simulink model "ResidentialPVArray"  (R2024b)
settings: Solver=FixedStepDiscrete  StartTime=0.0  StopTime=0.8  FixedStep=Ts_Power  RelTol=1e-4
PreLoadFcn:
  | Ts_Power=5e-6;
  | Ts_Control=25e-6;
  | Vf_Diode=0.6;
undefined symbols (not defined in the file or in its folder): DiscIntNeverNeededParam
libraries: spsDiodeLib x7, spsSeriesRLCLoadLib x6, spsPVArrayLib x6, spsVoltageMeasurementLib x5, spsSeriesRLCBranchLib x5, spsCurrentMeasurementLib x4, simulink x4, spsPowerLib x3, spsMeanLib x3, spsStairGeneratorLib x2, spsFirstOrderFilterLib x2, spsPWMGeneratorPulseAveragingLib x2
settings Model: SimulationMode=accelerator  Creator=The MathWorks, Inc.  LastModifiedBy=Jatay
settings SolverCC: AlgebraicLoopSolver=TrustRegion
settings DataIOCC: SaveFormat=StructureWithTime  SaveOutput=off  DSMLogging=off  SaveTime=off  ReturnWorkspaceOutputs=off
settings DebuggingCC: UnconnectedInputMsg=warning  UnconnectedOutputMsg=warning  UnconnectedLineMsg=warning  ArithmeticOperatorsInVariantConditions=warning
settings ModelReferenceCC: EnableRefExpFcnMdlSchedulingChecks=on
settings SFSimCC: CustomCodeUndefinedFunction=UseInterfaceOnly
settings RTWCC: GPUComputeCapability=3.5

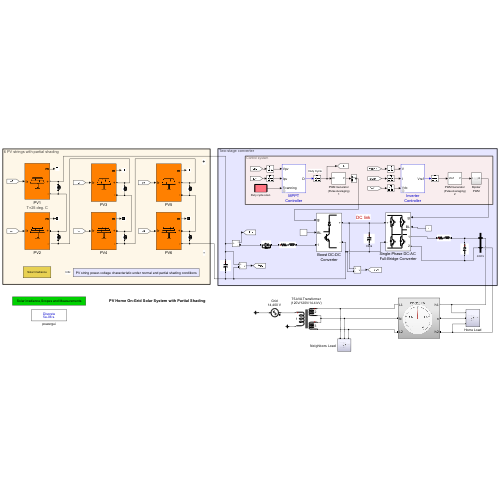
[thumbnail: Simulink's stored preview of the top-level diagram]
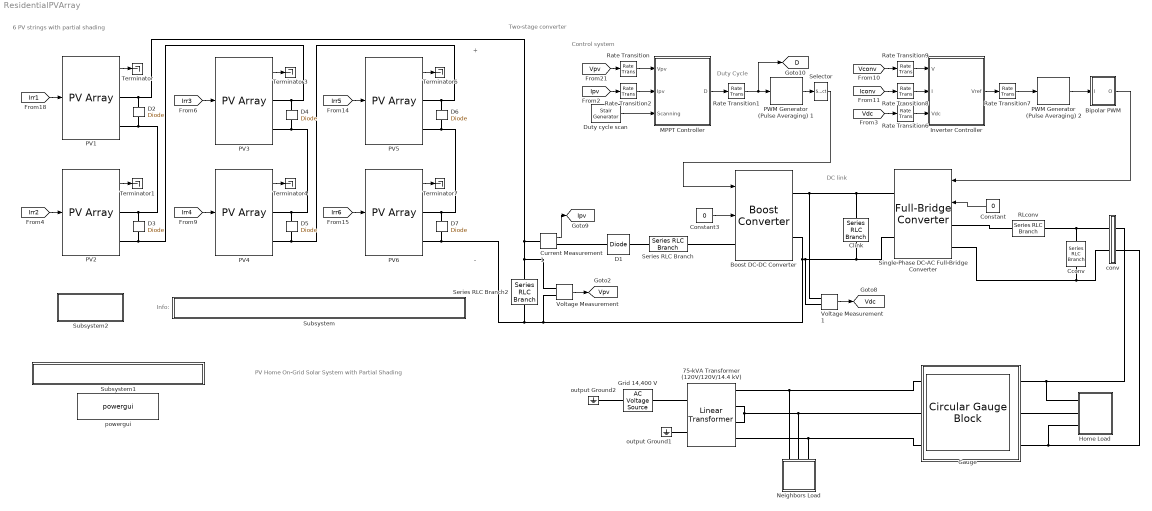
== system ResidentialPVArray ==
  note: Duty Cycle
  note: DC link
  note: Info:
  note: Control system
  note: Two-stage converter
  note: PV Home On-Grid Solar System with Partial Shading
  note: +
  note: 6 PV strings with partial shading
  note: -
  " " : Subsystem
  75-kVA Transformer (120V/120V/14.4 kV) : spsLinearTransformerLib/Linear Transformer  UNITS=pu  NominalPower=[75e3,60]  winding1=[14.4e3 0.01,0.03]  winding2=[120,0.02,0]  ThreeWindings=on  winding3=[120,0.02,0]  RmLm=[100,100]  Measurements=None  DataType=off
  Bipolar PWM : Subsystem
  Boost DC-DC Converter : spsBoostConverterLib/Boost Converter  ModelType=Switching function  Ron=1e-3  Rs=1e6  Cs=inf  Vforward=[0,0]  Ron_Diode=1e-3  Rs_Diode=1e6  Cs_Diode=inf  Vf_Diode=0  Rs_CurrentSource=inf  Ron_ACsource=1e-3
  Cconv : spsSeriesRLCBranchLib/Series RLC Branch  LConnTagsString=__new0  RConnTagsString=__new0  BranchType=C  Resistance=2  Inductance=10e-3  SetiL0=off  InitialCurrent=0  Capacitance=4e-6  Setx0=off  InitialVoltage=0  Measurements=None
  Clink : spsSeriesRLCBranchLib/Series RLC Branch  LConnTagsString=__new0  RConnTagsString=__new0  BranchType=C  Resistance=1e-6  Inductance=1e-3  SetiL0=off  InitialCurrent=0  Capacitance=5.0e-3  Setx0=on  InitialVoltage=400  Measurements=None
  Constant : Constant  Value=0
  Constant3 : Constant  Value=0
  Current Measurement1 : spsCurrentMeasurementLib/Current Measurement  PhasorSimulation=off  OutputType=Complex  PSBequivalent=0
  D{1..7} (7 alike) : spsDiodeLib/Diode  Ron=1e-3  Lon=0  Vf=Vf_Diode  IC=0  UseSnubber=0  Rs=1e6  Cs=inf  Measurements=off
  Duty cycle scan : spsStairGeneratorLib/Stair Generator  t=[0,0.40, 0.41]  e=[0, 1, 0]  Ts=Ts_Control
  Gauge : CircularGaugeBlock  ScaleMin=-3  ScaleMax=3  TickInterval=1.5
  Grid 14,400 V : spsACVoltageSourceLib/AC Voltage Source  Description=source block  Amplitude=14400*sqrt(2)  Phase=0  Frequency=60  SampleTime=0  Measurements=None  BusType=swing  Pref=10e3  Qref=0  Qmin=-inf  Qmax=+inf
      settings: AttributesFormatString=\n
  Home Load : Subsystem
  Inverter Controller : Subsystem  mask(Inverter Control){Pnom=2500, Fnom=60, Vnom_ac=240, Vnom_dc=400, Kp_VDCreg=10, Ki_VDCreg=1000, Kp_Ireg=0.3, Ki_Ireg=20, RLff=[ 0.003, 0.3], Ts=Ts_Control}
      mask prompts: Pnom "Power (VA)"; Fnom "Frequency (Hz)"; Vnom_ac "AC voltage (Vrms)"; Vnom_dc "DC voltage (V)"; Kp_VDCreg "Proportional gain"; Ki_VDCreg "Integral gain"; Kp_Ireg "Proportional gain"; Ki_Ireg "Integral gain"; RLff "Feedforward Values [Rff Lff] (pu)"; Ts "Control sample time:"
      mask help: Control system for a 2.5 kW Grid-Connected Inverter
      mask init:
      | Rff=RLff(1);
      | Lff=RLff(2);
      | Limits_Ireg=[1.5, -1.5];
      | Limits_VDCreg=[1.5, -1.5];
      | Limits_Preg=[1.5, -1.5];
      | Limits_Qreg=[1.5, -1.5];
      mask DialogControl Container4 Prompt: Nominal Values:
      mask DialogControl Container8 Prompt: Voltage regulator:
      mask DialogControl Container6 Prompt: Current regulators:
      mask DialogControl Ts1 Prompt: Sample time (s)
  MPPT Controller : Subsystem  mask(MPPT Controller - Perturb and Observe algorithm (PandO)){Dinit=0.39, Dlimits=[0.85, 0.30], deltaD=50e-6, Fc=1000, ScanDuration=0.25, Ts=Ts_Control}
      mask prompts: Dinit "Duty cycle (D) initial value"; Dlimits "D limits [Upper, Lower]"; deltaD "Increment value for PandO algorithm"; Fc "Measurement filter cutoff frequency (Hz)"; ScanDuration "Scanning mode duration (s)"; Ts "Sample time (s)"
      mask init:
      | Dmax=Dlimits(1);
      | Dmin=Dlimits(2);
      | SampleTime=Ts;
      | DeltaD_Scan=(Dmax-Dmin)*Ts/ScanDuration;
  Neighbors Load : Subsystem
  PV1 : spsPVArrayLib/PV Array  Npar=1  Nser=1  PlotType=array @ 25 deg.C & specified irradiances  S_vec=[ 1000 250]  Temp_C_vec="[ 45 25  ]"  ModuleName=User-defined  PlotWhenSelected=off  Pm=400.316  Ncell=72  Voc=49.3  Isc=10.47  Vm=40.6  Im=9.86  beta_Voc_pc=-0.2600  alpha_Isc_pc=0.03  beta_Voc=-0.12818  alpha_Isc=0.003141  IL=10.5166  I0=5.8445e-12  nI=0.94527  Rsh=194.9682  Rs=0.32878  RobustModel=on  RobustCellTemperature=25  BAL=on  Tc=1e-6  Tfilter=5e-5
      settings: AttributesFormatString=T=%<RobustCellTemperature> deg. C
  PV{2..6} (5 alike) : spsPVArrayLib/PV Array  Npar=1  Nser=1  PlotType=array @ 1000 W/m2 & specified temperatures  S_vec=[ 1000 250]  Temp_C_vec="[ 45 25  ]"  ModuleName=User-defined  PlotWhenSelected=off  Pm=400.316  Ncell=72  Voc=49.3  Isc=10.47  Vm=40.6  Im=9.86  beta_Voc_pc=-0.2600  alpha_Isc_pc=0.03  beta_Voc=-0.12818  alpha_Isc=0.003141  IL=10.5166  I0=5.8445e-12  nI=0.94527  Rsh=194.9682  Rs=0.32878  RobustModel=on  RobustCellTemperature=25  BAL=on  Tc=1e-6  Tfilter=5e-5
  PWM Generator (Pulse Averaging) 1 : spsPWMGeneratorPulseAveragingLib/PWM Generator (Pulse Averaging)  GeneratorType=Two-quadrant  Fc=20e3  InitialPhase=90  Ts=Ts_Power
  PWM Generator (Pulse Averaging) 2 : spsPWMGeneratorPulseAveragingLib/PWM Generator (Pulse Averaging)  GeneratorType=Full-bridge, single phase  Fc=20e3  InitialPhase=90  Ts=Ts_Power
  RLconv : spsSeriesRLCBranchLib/Series RLC Branch  LConnTagsString=__new0  RConnTagsString=__new0  BranchType=RL  Resistance=75e-3  Inductance=20e-3  SetiL0=off  InitialCurrent=0  Capacitance=1e-6  Setx0=off  InitialVoltage=0  Measurements=None
  Rate Transition{,2,6,8..9} (5 alike) : RateTransition  OutPortSampleTime=Ts_Control
  Rate Transition1 : RateTransition  OutPortSampleTime=Ts_Power
  Rate Transition7 : RateTransition  OutPortSampleTime=Ts_Power
  Selector : Selector  InputPortWidth=2  IndexOptions=Index vector (dialog)  Indices=1  OutputSizes=1
  Series RLC Branch : spsSeriesRLCBranchLib/Series RLC Branch  LConnTagsString=__new0  RConnTagsString=__new0  BranchType=RL  Resistance=20e-3  Inductance=20e-3  SetiL0=off  InitialCurrent=0  Capacitance=1e-6  Setx0=off  InitialVoltage=0  Measurements=None
  Series RLC Branch2 : spsSeriesRLCBranchLib/Series RLC Branch  LConnTagsString=__new0  RConnTagsString=__new0  BranchType=C  Resistance=10e-3  Inductance=10e-3  SetiL0=off  InitialCurrent=0  Capacitance=10e-6  Setx0=off  InitialVoltage=0  Measurements=None
  Single-Phase DC-AC Full-Bridge Converter : spsFullBridgeConverterLib/Full-Bridge Converter  ModelType=Switching function  Ron=1e-3  Rs=1e6  Cs=inf  Vforward=[0,0]  Ron_Diode=1e-3  Rs_Diode=1e6  Cs_Diode=inf  Vf_Diode=0  Rs_CurrentSource=inf  Ron_ACsource=1e-3
  Subsystem : Subsystem
      mask Display: disp('PV string power-voltage characteristic under normal and partial shading conditions')
  Subsystem1 : Subsystem
      mask Display: disp('Solar irradiance,Scopes and Measurements')
  Subsystem2 : Subsystem
      mask Display: disp('Solar Irradiance')
  Terminator{,1,3..4,6..7} (6 alike) : Terminator
  Voltage Measurement : spsVoltageMeasurementLib/Voltage Measurement  PhasorSimulation=off  OutputType=Complex  PSBequivalent=0
  Voltage Measurement1 : spsVoltageMeasurementLib/Voltage Measurement  PhasorSimulation=off  OutputType=Complex  PSBequivalent=0
  conv : Subsystem
  output Ground1 : spsGroundLib/Ground  LConnTagsString=a
  output Ground2 : spsGroundLib/Ground  LConnTagsString=a
  powergui : spspowerguiLib/powergui  Priority=2  SimulationMode=Discrete  SampleTime=Ts_Power  frequency=60  Iterations=50  frequencyindice=0  Pbase=100e6  ErrMax=1e-4  UnitsV=kV  UnitsW=MW  buscounter=0  FunctionMessages=off  echomessages=off  EnableUseOfTLC=off  CurrentSourceSwitches=off  DisableSnubberDevices=off  DisableRonSwitches=off  DisableVfSwitches=off  DisplayEquations=off  AutomaticDiscreteSolvers=off  SolverType=Tustin/Backward Euler (TBE)  Interpol=off  ExternalGateDelay=off  methode=off  Ts=0  x0status=blocks  SPID=off  SwTol=0  HookPort=off  NonlinearTolerance=1e-4  nMaxIteration=100  ContinueOnMaxIteration=on  RestoreLinks=warning  ResistiveCurrentMeasurement=off  Frange=[0:2:500]  Ylog=off  Xlog=off  ShowGrid=off  save=off  variable=ZData  structure=Scope_VIgrid  ZoomFFT=off  StartTime=0.27  cycles=1  DisplayStyle=1  fundamental=60  FreqAxis=off  MaxFrequency=25000  frequencyindicesteady=1  RmsSteady=1  display=off
  tag scope: D=global, Ipv=global, Vdc=global, Vpv=global
  wires:
  [Irr1] -> PV1/1
  MPPT Controller/1(D) -> Rate Transition1/1
  PV1/1 -> Terminator/1
  [Irr2] -> PV2/1
  PV2/1 -> Terminator1/1
  [Irr3] -> PV3/1
  PV3/1 -> Terminator3/1
  PV4/1 -> Terminator4/1
  [Irr4] -> PV4/1
  PV6/1 -> Terminator7/1
  PV5/1 -> Terminator6/1
  [Irr6] -> PV6/1
  [Irr5] -> PV5/1
  Voltage Measurement/1 -> [Vpv]
  Constant3/1 -> Boost DC-DC Converter/2
  Duty cycle scan/1 -> MPPT Controller/3(Scanning)
  [Ipv] -> Rate Transition2/1
  [Vpv] -> Rate Transition/1
  Rate Transition/1 -> MPPT Controller/1(Vpv)
  Rate Transition2/1 -> MPPT Controller/2(Ipv)
  [Vconv] -> Rate Transition9/1
  [Vdc] -> Rate Transition6/1
  [Iconv] -> Rate Transition8/1
  Rate Transition6/1 -> Inverter Controller/3(Vdc)
  Rate Transition8/1 -> Inverter Controller/2(I)
  Rate Transition9/1 -> Inverter Controller/1(V)
  Voltage Measurement1/1 -> [Vdc]
  Constant/1 -> Single-Phase DC-AC Full-Bridge Converter/2
  Current Measurement1/1 -> [Ipv]
  Rate Transition7/1 -> PWM Generator (Pulse Averaging) 2/1
  Inverter Controller/1(Vref) -> Rate Transition7/1
  Rate Transition1/1 -> PWM Generator (Pulse Averaging) 1/1, [D]
  Selector/1 -> Boost DC-DC Converter/1
  PWM Generator (Pulse Averaging) 1/1 -> Selector/1
  PWM Generator (Pulse Averaging) 2/1 -> Bipolar PWM/1(I)
  Bipolar PWM/1(O) -> Single-Phase DC-AC Full-Bridge Converter/1
  connections:
  PV5/RConn1 -- D5/LConn1 -- PV4/RConn2 -- D6/RConn1
  D2/LConn1 -- D3/RConn1 -- PV2/RConn1 -- PV1/RConn2
  D4/RConn1 -- D3/LConn1 -- PV2/RConn2 -- PV3/RConn1
  D4/LConn1 -- D5/RConn1 -- PV4/RConn1 -- PV3/RConn2
  D6/LConn1 -- D7/RConn1 -- PV6/RConn1 -- PV5/RConn2
  D1/RConn1 -- Series RLC Branch/LConn1
  Series RLC Branch/RConn1 -- Boost DC-DC Converter/LConn1
  D7/LConn1 -- PV6/RConn2 -- Series RLC Branch2/RConn1 -- Voltage Measurement/LConn2 -- Clink/RConn1 -- Single-Phase DC-AC Full-Bridge Converter/RConn2 -- Voltage Measurement1/LConn2 -- Boost DC-DC Converter/RConn2
  Clink/LConn1 -- Single-Phase DC-AC Full-Bridge Converter/RConn1 -- Voltage Measurement1/LConn1 -- Boost DC-DC Converter/RConn1
  Current Measurement1/RConn1 -- D1/LConn1
  75-kVA Transformer (120V/120V/14.4 kV)/RConn2 -- " "/RConn2 -- Neighbors Load/LConn2 -- 75-kVA Transformer (120V/120V/14.4 kV)/RConn3
  output Ground2/LConn1 -- Grid 14,400 V/LConn1
  Single-Phase DC-AC Full-Bridge Converter/LConn1 -- RLconv/LConn1
  Grid 14,400 V/RConn1 -- 75-kVA Transformer (120V/120V/14.4 kV)/LConn1
  Single-Phase DC-AC Full-Bridge Converter/LConn2 -- Cconv/RConn1 -- conv/LConn2
  RLconv/RConn1 -- Cconv/LConn1 -- conv/LConn1
  Voltage Measurement/LConn1 -- D2/RConn1 -- PV1/RConn1 -- Current Measurement1/LConn1 -- Series RLC Branch2/LConn1
  " "/RConn1 -- Neighbors Load/LConn1 -- 75-kVA Transformer (120V/120V/14.4 kV)/RConn1
  Home Load/LConn1 -- conv/RConn1 -- " "/LConn1
  conv/RConn2 -- Home Load/LConn3 -- " "/LConn3
  " "/RConn3 -- Neighbors Load/LConn3 -- 75-kVA Transformer (120V/120V/14.4 kV)/RConn4
  Home Load/LConn2 -- " "/LConn2
  output Ground1/LConn1 -- 75-kVA Transformer (120V/120V/14.4 kV)/LConn2

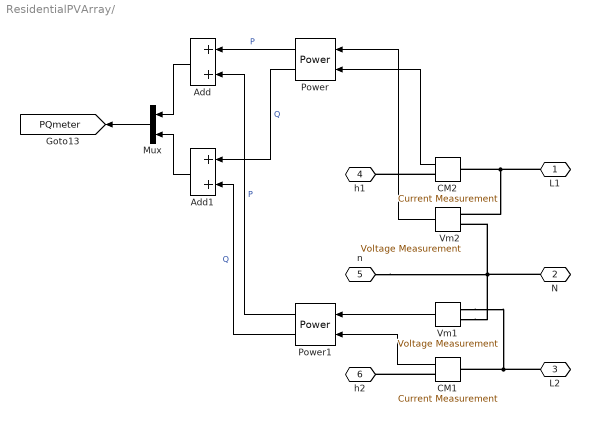
== system ResidentialPVArray/  ==
  Add : Sum
  Add1 : Sum
  CM1 : spsCurrentMeasurementLib/Current Measurement  PhasorSimulation=off  OutputType=Complex  PSBequivalent=0
  CM2 : spsCurrentMeasurementLib/Current Measurement  PhasorSimulation=off  OutputType=Complex  PSBequivalent=0
  Mux : Mux  Inputs=2
  Power : spsPowerLib/Power  Freq=60  Vinit=[120*sqrt(2), 0]*0  Iinit=[10*sqrt(2), 10]*0  Ts=Ts_Power
  Power1 : spsPowerLib/Power  Freq=60  Vinit=[120*sqrt(2), 0]*0  Iinit=[10*sqrt(2), 10]*0  Ts=Ts_Power
  Vm1 : spsVoltageMeasurementLib/Voltage Measurement  PhasorSimulation=off  OutputType=Complex  PSBequivalent=0
  Vm2 : spsVoltageMeasurementLib/Voltage Measurement  PhasorSimulation=off  OutputType=Complex  PSBequivalent=0
  L1 : PMIOPort  Side=Right
  N : PMIOPort  Port=2  Side=Right
  L2 : PMIOPort  Port=3  Side=Right
  h1 : PMIOPort  Port=4  Side=Left
  n : PMIOPort  Port=5  Side=Left
  h2 : PMIOPort  Port=6  Side=Left
  tag scope: PQmeter=global
  wires:
  Vm2/1 -> Power/1
  CM2/1 -> Power/2
  Vm1/1 -> Power1/1
  CM1/1 -> Power1/2
  Power/1 -> Add/1  "P"
  Power1/1 -> Add/2  "P"
  Add/1 -> Mux/1
  Power/2 -> Add1/1  "Q"
  Power1/2 -> Add1/2  "Q"
  Add1/1 -> Mux/2
  Mux/1 -> [PQmeter]
  connections:
  Vm1/LConn2 -- N/RConn1 -- n/RConn1 -- Vm2/LConn2
  Vm2/LConn1 -- L1/RConn1 -- CM2/LConn1
  CM2/RConn1 -- h1/RConn1
  L2/RConn1 -- Vm1/LConn1 -- CM1/LConn1
  CM1/RConn1 -- h2/RConn1

== system ResidentialPVArray/Bipolar PWM ==
  I : Inport
  Demux : Demux
  Mux : Mux
  Terminator : Terminator
  Terminator1 : Terminator
  O : Outport  VectorParamsAs1DForOutWhenUnconnected=off
  wires:
  Demux/4 -> Terminator1/1
  Demux/3 -> Terminator/1
  Demux/2 -> Mux/2, Mux/3
  Demux/1 -> Mux/1, Mux/4
  I/1 -> Demux/1
  Mux/1 -> O/1

== system ResidentialPVArray/Home Load ==
  HomeLoad 120V_1 : spsSeriesRLCLoadLib/Series RLC Load  LConnTagsString=a  RConnTagsString=__new0  NominalVoltage=120  NominalFrequency=60  ActivePower=600  InductivePower=0  CapacitivePower=0  Setx0=off  InitialVoltage=0  SetiL0=off  InitialCurrent=0  Measurements=None  LoadType=constant Z
  HomeLoad 120V_2 : spsSeriesRLCLoadLib/Series RLC Load  LConnTagsString=a  RConnTagsString=__new0  NominalVoltage=120  NominalFrequency=60  ActivePower=400  InductivePower=0  CapacitivePower=0  Setx0=off  InitialVoltage=0  SetiL0=off  InitialCurrent=0  Measurements=None  LoadType=constant Z
  HomeLoad 240V : spsSeriesRLCLoadLib/Series RLC Load  LConnTagsString=a  RConnTagsString=__new0  NominalVoltage=240  NominalFrequency=60  ActivePower=1.5e3  InductivePower=250  CapacitivePower=0  Setx0=off  InitialVoltage=0  SetiL0=off  InitialCurrent=0  Measurements=None  LoadType=constant Z
  R : PMIOPort  Side=Left
  W : PMIOPort  Port=2  Side=Left
  B : PMIOPort  Port=3  Side=Left
  connections:
  HomeLoad 120V_1/RConn1 -- R/RConn1 -- HomeLoad 240V/RConn1
  HomeLoad 120V_2/RConn1 -- W/RConn1 -- HomeLoad 120V_1/LConn1
  HomeLoad 120V_2/LConn1 -- B/RConn1 -- HomeLoad 240V/LConn1

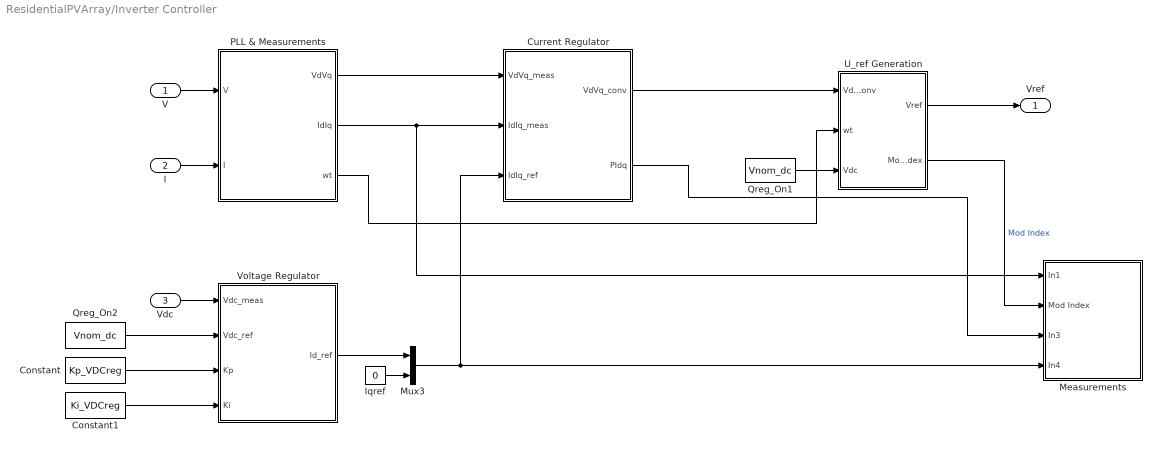
== system ResidentialPVArray/Inverter Controller ==
  V : Inport  PortDimensions=1
  I : Inport  Port=2  PortDimensions=1
  Vdc : Inport  Port=3  PortDimensions=1
  Constant : Constant  Value=Kp_VDCreg  SampleTime=Ts
  Constant1 : Constant  Value=Ki_VDCreg  SampleTime=Ts
  Current Regulator : Subsystem
  Iqref : Constant  Value=0  SampleTime=Ts
  Measurements : Subsystem
  Mux3 : Mux  Inputs=2
  PLL & Measurements : Subsystem
  Qreg_On1 : Constant  Value=Vnom_dc
  Qreg_On2 : Constant  Value=Vnom_dc
  "U_ref Generation " : Subsystem
  Voltage Regulator : Subsystem
  Vref : Outport  VectorParamsAs1DForOutWhenUnconnected=off
  wires:
  Constant/1 -> Voltage Regulator/3(Kp)
  Mux3/1 -> Current Regulator/3(IdIq_ref), Measurements/4(In4)
  V/1 -> PLL & Measurements/1(V)
  Qreg_On2/1 -> Voltage Regulator/2(Vdc_ref)
  PLL & Measurements/2(IdIq) -> Measurements/1(In1), Current Regulator/2(IdIq_meas)
  Voltage Regulator/1(Id_ref) -> Mux3/1
  Constant1/1 -> Voltage Regulator/4(Ki)
  Iqref/1 -> Mux3/2
  I/1 -> PLL & Measurements/2(I)
  Vdc/1 -> Voltage Regulator/1(Vdc_meas)
  PLL & Measurements/1(VdVq) -> Current Regulator/1(VdVq_meas)
  "U_ref Generation "/1(Vref) -> Vref/1
  PLL & Measurements/3(wt) -> "U_ref Generation "/2(wt)
  Qreg_On1/1 -> "U_ref Generation "/3(Vdc)
  Current Regulator/1(VdVq_conv) -> "U_ref Generation "/1(VdVq_conv)
  "U_ref Generation "/2(ModIndex) -> Measurements/2(Mod Index)  "Mod Index"
  Current Regulator/2(PIdq) -> Measurements/3(In3)

== system ResidentialPVArray/MPPT Controller ==
  note: D = 1 - Vsrc/Vdc
  Vpv : Inport
  Ipv : Inport  Port=2
  Scanning : Inport  Port=3  PortDimensions=1
  First-Order Filter : spsFirstOrderFilterLib/First-Order Filter  FilterType=Lowpass  Tc=1/Fc  Ts=Ts  Initialize=off  Vac_Init=[0, 0, 60]  Vdc_Init=0  PlotResponse=off  FreqRange="[0,  200,  1]"
  First-Order Filter1 : spsFirstOrderFilterLib/First-Order Filter  FilterType=Lowpass  Tc=1/Fc  Ts=Ts  Initialize=off  Vac_Init=[0, 0, 60]  Vdc_Init=0  PlotResponse=off  FreqRange="[0,  200,  1]"
  MPPT Control : MATLAB Function  TreatAsAtomicUnit=on
  D : Outport  OutDataTypeStr=double  PortDimensions=1  VectorParamsAs1DForOutWhenUnconnected=off
  wires:
  First-Order Filter1/1 -> MPPT Control/2(I)
  First-Order Filter/1 -> MPPT Control/1(V)
  Ipv/1 -> First-Order Filter1/1
  Vpv/1 -> First-Order Filter/1
  MPPT Control/1(D) -> D/1
  Scanning/1 -> MPPT Control/3(Scan_On)

== system ResidentialPVArray/Neighbors Load ==
  Load 120V_1 : spsSeriesRLCLoadLib/Series RLC Load  LConnTagsString=a  RConnTagsString=__new0  NominalVoltage=120  NominalFrequency=60  ActivePower=7e3  InductivePower=0  CapacitivePower=0  Setx0=off  InitialVoltage=0  SetiL0=off  InitialCurrent=0  Measurements=None  LoadType=constant Z
  Load 120V_2 : spsSeriesRLCLoadLib/Series RLC Load  LConnTagsString=a  RConnTagsString=__new0  NominalVoltage=120  NominalFrequency=60  ActivePower=4e3  InductivePower=0  CapacitivePower=0  Setx0=off  InitialVoltage=0  SetiL0=off  InitialCurrent=0  Measurements=None  LoadType=constant Z
  Load 240V : spsSeriesRLCLoadLib/Series RLC Load  LConnTagsString=a  RConnTagsString=__new0  NominalVoltage=240  NominalFrequency=60  ActivePower=15e3  InductivePower=2000  CapacitivePower=0  Setx0=off  InitialVoltage=0  SetiL0=off  InitialCurrent=0  Measurements=None  LoadType=constant Z
  R : PMIOPort  Side=Left
  W : PMIOPort  Port=2  Side=Left
  B : PMIOPort  Port=3  Side=Left
  connections:
  B/RConn1 -- Load 120V_2/LConn1 -- Load 240V/LConn1
  W/RConn1 -- Load 120V_2/RConn1 -- Load 120V_1/LConn1
  R/RConn1 -- Load 120V_1/RConn1 -- Load 240V/RConn1

== system ResidentialPVArray/Subsystem ==
  note: 6 * LG Electronics Inc. LG400N2W-A5

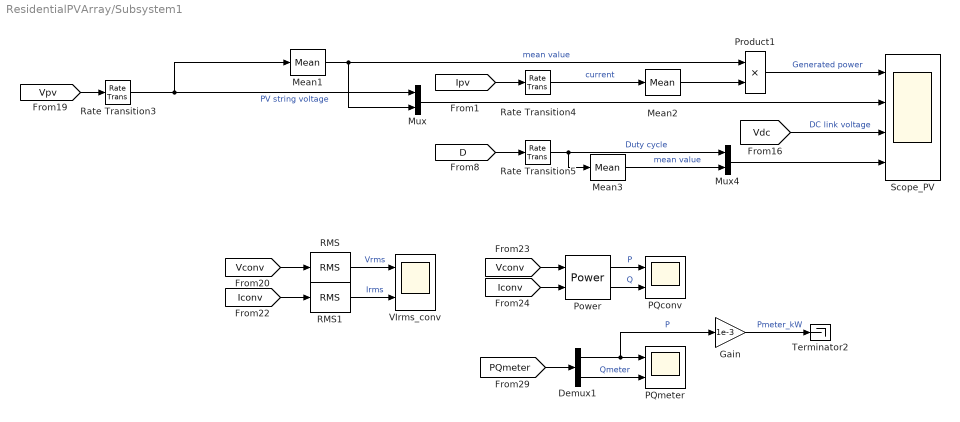
== system ResidentialPVArray/Subsystem1 ==
  Demux1 : Demux  Outputs=2
  Gain : Gain  Gain=1e-3
  Mean1 : spsMeanLib/Mean  Freq=60  Vinit=250  Ts=Ts_Control
  Mean2 : spsMeanLib/Mean  Freq=60  Vinit=10  Ts=Ts_Control
  Mean3 : spsMeanLib/Mean  Freq=60  Vinit=0.4  Ts=Ts_Control
  Mux : Mux  Inputs=2
  Mux4 : Mux  Inputs=2
  PQconv : Scope  NumInputPorts=2
  PQmeter : Scope  NumInputPorts=2
  Power : spsPowerLib/Power  Freq=60  Vinit=[240*sqrt(2), 0]  Iinit=[10*sqrt(2), 10]  Ts=Ts_Power
  Product1 : Product
  RMS : spsRMSLib/RMS  TrueRMS=on  Freq=60  RMSInit=240  Ts=Ts_Power
  RMS1 : spsRMSLib/RMS  TrueRMS=on  Freq=60  RMSInit=10  Ts=Ts_Power
  Rate Transition3 : RateTransition  OutPortSampleTime=Ts_Control
  Rate Transition4 : RateTransition  OutPortSampleTime=Ts_Control
  Rate Transition5 : RateTransition  OutPortSampleTime=Ts_Control
  Scope_PV : Scope  NumInputPorts=4
  Terminator2 : Terminator
  VIrms_conv : Scope  NumInputPorts=2
  wires:
  Gain/1 -> Terminator2/1  "Pmeter_kW"
  [D] -> Rate Transition5/1
  Rate Transition5/1 -> Mean3/1, Mux4/1  "Duty cycle"
  Mean3/1 -> Mux4/2  "mean value"
  Mux4/1 -> Scope_PV/4
  Demux1/2 -> PQmeter/2  "Qmeter"
  [PQmeter] -> Demux1/1
  Demux1/1 -> PQmeter/1, Gain/1  "P"
  [Vconv] -> Power/1
  [Iconv] -> Power/2
  [Iconv] -> RMS1/1
  [Vconv] -> RMS/1
  RMS1/1 -> VIrms_conv/2  "Irms"
  Power/2 -> PQconv/2  "Q"
  Power/1 -> PQconv/1  "P"
  RMS/1 -> VIrms_conv/1  "Vrms"
  [Vdc] -> Scope_PV/3  "DC link voltage"
  Product1/1 -> Scope_PV/1  "Generated power"
  Mux/1 -> Scope_PV/2
  Rate Transition4/1 -> Mean2/1  "current"
  Rate Transition3/1 -> Mean1/1, Mux/1  "PV string voltage"
  Mean2/1 -> Product1/2
  Mean1/1 -> Mux/2, Product1/1  "mean value"
  [Ipv] -> Rate Transition4/1
  [Vpv] -> Rate Transition3/1

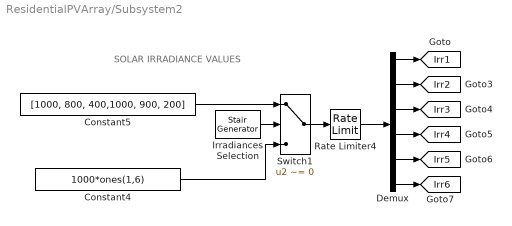
== system ResidentialPVArray/Subsystem2 ==
  note: SOLAR IRRADIANCE VALUES
  Constant4 : Constant  Value=1000*ones(1,6)
  Constant5 : Constant  Value=[1000, 800, 400,1000, 900, 200]
  Demux : Demux  Outputs=6
  Irradiances Selection : spsStairGeneratorLib/Stair Generator  t=[0,0.3, 1.3]  e=[0, 1, 0]  Ts=Ts_Power
  Rate Limiter4 : RateLimiter  RisingSlewLimit=1000*60  FallingSlewLimit=-1000*60  SampleTimeMode=inherited  InitialCondition=1000
  Switch1 : Switch  Criteria=u2 ~= 0  SaturateOnIntegerOverflow=off  InputSameDT=off
  tag scope: Irr1=global, Irr2=global, Irr3=global, Irr4=global, Irr5=global, Irr6=global
  wires:
  Constant5/1 -> Switch1/1
  Demux/5 -> [Irr5]
  Constant4/1 -> Switch1/3
  Irradiances Selection/1 -> Switch1/2
  Rate Limiter4/1 -> Demux/1
  Demux/1 -> [Irr1]
  Switch1/1 -> Rate Limiter4/1
  Demux/3 -> [Irr3]
  Demux/6 -> [Irr6]
  Demux/2 -> [Irr2]
  Demux/4 -> [Irr4]

== system ResidentialPVArray/conv ==
  CM2 : spsCurrentMeasurementLib/Current Measurement  PhasorSimulation=off  OutputType=Complex  PSBequivalent=0
  Vm2 : spsVoltageMeasurementLib/Voltage Measurement  PhasorSimulation=off  OutputType=Complex  PSBequivalent=0
  A : PMIOPort  Side=Left
  B : PMIOPort  Port=2  Side=Left
  a : PMIOPort  Port=3  Side=Right
  b : PMIOPort  Port=4  Side=Right
  tag scope: Iconv=global, Vconv=global
  wires:
  CM2/1 -> [Iconv]
  Vm2/1 -> [Vconv]
  connections:
  CM2/RConn1 -- a/RConn1
  CM2/LConn1 -- A/RConn1 -- Vm2/LConn1
  B/RConn1 -- b/RConn1 -- Vm2/LConn2

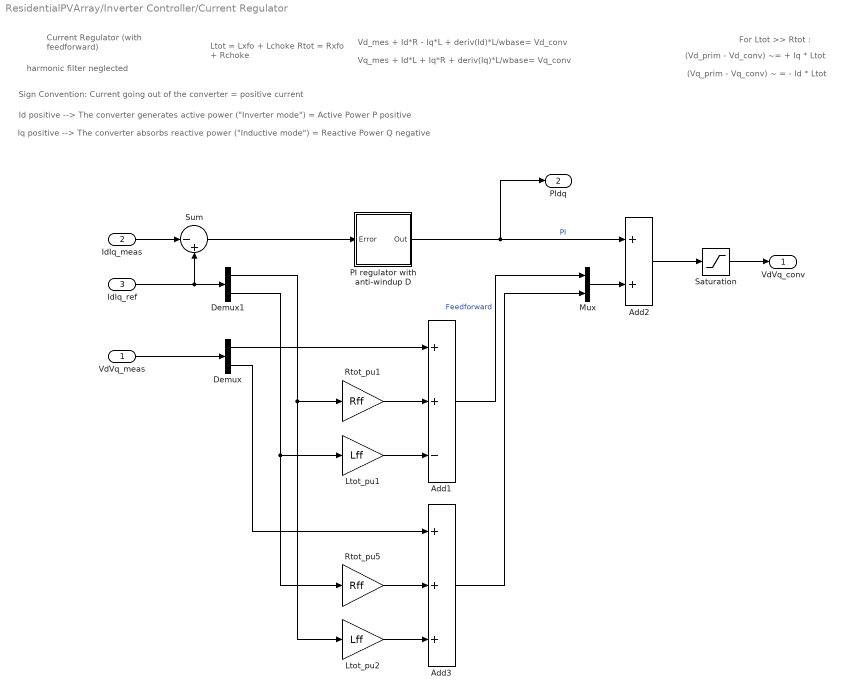
== system ResidentialPVArray/Inverter Controller/Current Regulator ==
  note: harmonic filter neglected
  note: Vd_mes + Id*R - Iq*L + deriv(Id)*L/wbase= Vd_conv
  note: Vq_mes + Id*L + Iq*R + deriv(Iq)*L/wbase= Vq_conv
  note: Current Regulator
      | (with feedforward)
  note: Sign Convention: Current going out of the converter = positive current
  note: Iq positive --> The converter absorbs reactive power ("Inductive mode") = Reactive Power Q negative
  note: Id positive --> The converter generates active power ("Inverter mode") = Active Power P positive
  note: Ltot = Lxfo + Lchoke
      | Rtot = Rxfo + Rchoke
  note: (Vd_prim - Vd_conv) ~= + Iq * Ltot
  note: (Vq_prim - Vq_conv) ~ = - Id * Ltot
  note: For Ltot >> Rtot :
  VdVq_meas : Inport  PortDimensions=2
  IdIq_meas : Inport  Port=2  PortDimensions=2
  IdIq_ref : Inport  Port=3  PortDimensions=2
  Add1 : Sum  Inputs=++-
  Add2 : Sum
  Add3 : Sum  Inputs=+++
  Demux : Demux  Outputs=2
  Demux1 : Demux  Outputs=2
  Ltot_pu1 : Gain  Gain=Lff  SaturateOnIntegerOverflow=on  OutDataTypeStr=Inherit: Same as input  ParamDataTypeStr=Inherit: Same as input
  Ltot_pu2 : Gain  Gain=Lff  SaturateOnIntegerOverflow=on  OutDataTypeStr=Inherit: Same as input  ParamDataTypeStr=Inherit: Same as input
  Mux : Mux  Inputs=2
  PI regulator with anti-windup D : Subsystem  DialogController=POWERSYS.PowerSysDialog  mask(Discrete PI Controller){Kp=Kp_Ireg, Ki=Ki_Ireg, Par_Limits=Limits_Ireg, Init=0, Ts=Ts}
      mask prompts: Kp "Proportional gain (Kp):"; Ki "Integral gain (Ki):"; Par_Limits "Output limits: [ Upper   Lower ]"; Init "Output initial value:"; Ts "Sample time:"
      mask help: This block implements a discrete PI controller.
      mask init:
      | UpperLimit=Par_Limits(1);
      | LowerLimit=Par_Limits(2);
      | power_initmask();
      mask Help: This block is part of a subset of blocks in the Extras library that does not have documentation associated with it, other than the block mask description.
      mask Display: disp('PI');
  Rtot_pu1 : Gain  Gain=Rff  SaturateOnIntegerOverflow=on  OutDataTypeStr=Inherit: Same as input  ParamDataTypeStr=Inherit: Same as input
  Rtot_pu5 : Gain  Gain=Rff  SaturateOnIntegerOverflow=on  OutDataTypeStr=Inherit: Same as input  ParamDataTypeStr=Inherit: Same as input
  Saturation : Saturate  UpperLimit=Limits_Ireg(1)  LowerLimit=Limits_Ireg(2)
  Sum : Sum  Inputs=|-+
  VdVq_conv : Outport  VectorParamsAs1DForOutWhenUnconnected=off
  PIdq : Outport  Port=2  VectorParamsAs1DForOutWhenUnconnected=off
  wires:
  Mux/1 -> Add2/2
  PI regulator with anti-windup D/1(Out) -> PIdq/1, Add2/1  "PI"
  Sum/1 -> PI regulator with anti-windup D/1(Error)
  IdIq_ref/1 -> Sum/2, Demux1/1
  IdIq_meas/1 -> Sum/1
  Add2/1 -> Saturation/1
  Saturation/1 -> VdVq_conv/1
  VdVq_meas/1 -> Demux/1
  Demux/1 -> Add1/1
  Rtot_pu1/1 -> Add1/2
  Demux1/1 -> Rtot_pu1/1, Ltot_pu2/1
  Ltot_pu1/1 -> Add1/3
  Demux1/2 -> Ltot_pu1/1, Rtot_pu5/1
  Rtot_pu5/1 -> Add3/2
  Ltot_pu2/1 -> Add3/3
  Add1/1 -> Mux/1  "Feedforward"
  Demux/2 -> Add3/1
  Add3/1 -> Mux/2

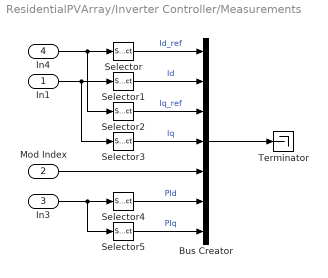
== system ResidentialPVArray/Inverter Controller/Measurements ==
  In1 : Inport
  Mod Index : Inport  Port=2
  In3 : Inport  Port=3
  In4 : Inport  Port=4
  Bus Creator : BusCreator  Inputs=7
  Selector : Selector  InputPortWidth=2  IndexOptions=Index vector (dialog)  Indices=1  OutputSizes=1
  Selector1 : Selector  InputPortWidth=2  IndexOptions=Index vector (dialog)  Indices=1  OutputSizes=1
  Selector2 : Selector  InputPortWidth=2  IndexOptions=Index vector (dialog)  Indices=2  OutputSizes=1
  Selector3 : Selector  InputPortWidth=2  IndexOptions=Index vector (dialog)  Indices=2  OutputSizes=1
  Selector4 : Selector  InputPortWidth=2  IndexOptions=Index vector (dialog)  Indices=1  OutputSizes=1
  Selector5 : Selector  InputPortWidth=2  IndexOptions=Index vector (dialog)  Indices=2  OutputSizes=1
  Terminator : Terminator
  wires:
  Selector3/1 -> Bus Creator/4  "Iq"
  Selector1/1 -> Bus Creator/2  "Id"
  In3/1 -> Selector5/1, Selector4/1
  In4/1 -> Selector/1, Selector2/1
  Selector2/1 -> Bus Creator/3  "Iq_ref"
  Selector5/1 -> Bus Creator/7  "PIq"
  Selector4/1 -> Bus Creator/6  "PId"
  Selector/1 -> Bus Creator/1  "Id_ref"
  In1/1 -> Selector1/1, Selector3/1
  Bus Creator/1 -> Terminator/1
  Mod Index/1 -> Bus Creator/5

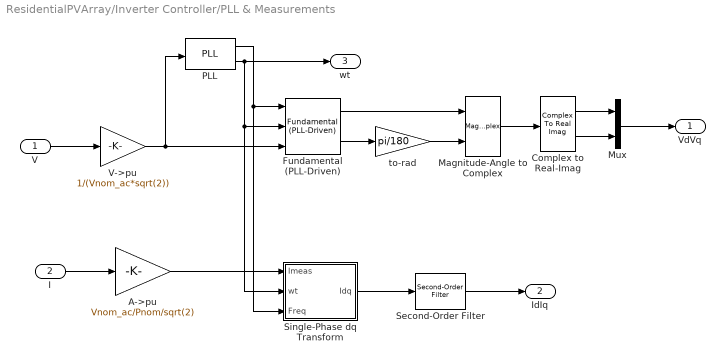
== system ResidentialPVArray/Inverter Controller/PLL & Measurements ==
  V : Inport
  I : Inport  Port=2
  A->pu : Gain  Gain=Vnom_ac/Pnom/sqrt(2)  SaturateOnIntegerOverflow=on  OutDataTypeStr=Inherit: Same as input  ParamDataTypeStr=Inherit: Same as input
  Complex to Real-Imag : ComplexToRealImag
  Fundamental (PLL-Driven) : spsFundamentalPLLDrivenLib/Fundamental (PLL-Driven)  Finit=Fnom  Fmin=45  InInit=[1, 0]  Ts=Ts
  Magnitude-Angle to Complex : MagnitudeAngleToComplex
  Mux : Mux  Inputs=2
  PLL : spsPLLLib/PLL  Fmin=45  Par_Init=[0, Fnom]  ParK=[180, 3200, 1]  TcD=1e-4  MaxRateChangeFreq=12  FilterCutOffFreq=25  Ts=Ts  AGC=on
  Second-Order Filter : spsSecondOrderFilterLib/Second-Order Filter  FilterType=Lowpass  Fo=2000  Zeta=1  Ts=Ts  Initialize=on  Vac_Init="[0,  0,  60;0,0,60]"  Vdc_Init=[0.9 0]  PlotResponse=off  FreqRange=[0, 500, 1]
  Single-Phase dq Transform : Subsystem
  V->pu : Gain  Gain=1/(Vnom_ac*sqrt(2))  SaturateOnIntegerOverflow=on  OutDataTypeStr=Inherit: Same as input  ParamDataTypeStr=Inherit: Same as input
  to-rad : Gain  Gain=pi/180
  VdVq : Outport  VectorParamsAs1DForOutWhenUnconnected=off
  IdIq : Outport  Port=2  VectorParamsAs1DForOutWhenUnconnected=off
  wt : Outport  Port=3  VectorParamsAs1DForOutWhenUnconnected=off
  wires:
  Second-Order Filter/1 -> IdIq/1
  Single-Phase dq Transform/1(Idq) -> Second-Order Filter/1
  V->pu/1 -> PLL/1, Fundamental (PLL-Driven)/3
  V/1 -> V->pu/1
  I/1 -> A->pu/1
  PLL/2 -> Single-Phase dq Transform/2(wt), Fundamental (PLL-Driven)/2, wt/1
  PLL/1 -> Fundamental (PLL-Driven)/1, Single-Phase dq Transform/3(Freq)
  A->pu/1 -> Single-Phase dq Transform/1(Imeas)
  Fundamental (PLL-Driven)/1 -> Magnitude-Angle to Complex/1
  Fundamental (PLL-Driven)/2 -> to-rad/1
  Magnitude-Angle to Complex/1 -> Complex to Real-Imag/1
  Complex to Real-Imag/1 -> Mux/1
  Complex to Real-Imag/2 -> Mux/2
  Mux/1 -> VdVq/1
  to-rad/1 -> Magnitude-Angle to Complex/2

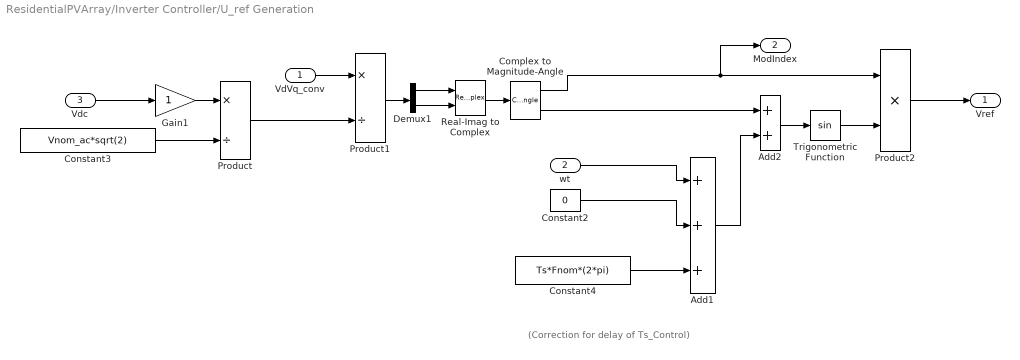
== system ResidentialPVArray/Inverter Controller/U_ref Generation  ==
  note: (Correction for delay of Ts_Control)
  VdVq_conv : Inport
  wt : Inport  Port=2
  Vdc : Inport  Port=3
  Add1 : Sum  Inputs=+++
  Add2 : Sum
  Complex to Magnitude-Angle : ComplexToMagnitudeAngle
  Constant2 : Constant  Value=0
  Constant3 : Constant  Value=Vnom_ac*sqrt(2)
  Constant4 : Constant  Value=Ts*Fnom*(2*pi)
  Demux1 : Demux  Outputs=2
  Gain1 : Gain
  Product : Product  Inputs=*/  RndMeth=Zero
  Product1 : Product  Inputs=*/  RndMeth=Zero
  Product2 : Product  Inputs=**  RndMeth=Zero
  Real-Imag to Complex : RealImagToComplex
  Trigonometric Function : Trigonometry
  Vref : Outport  VectorParamsAs1DForOutWhenUnconnected=off
  ModIndex : Outport  Port=2  VectorParamsAs1DForOutWhenUnconnected=off
  wires:
  Product1/1 -> Demux1/1
  Gain1/1 -> Product/1
  Real-Imag to Complex/1 -> Complex to Magnitude-Angle/1
  Demux1/1 -> Real-Imag to Complex/1
  Demux1/2 -> Real-Imag to Complex/2
  Constant2/1 -> Add1/2
  Constant3/1 -> Product/2
  Product/1 -> Product1/2
  Complex to Magnitude-Angle/2 -> Add2/1
  Add1/1 -> Add2/2
  Add2/1 -> Trigonometric Function/1
  Complex to Magnitude-Angle/1 -> ModIndex/1, Product2/1
  Trigonometric Function/1 -> Product2/2
  wt/1 -> Add1/1
  Constant4/1 -> Add1/3
  Vdc/1 -> Gain1/1
  Product2/1 -> Vref/1
  VdVq_conv/1 -> Product1/1

== system ResidentialPVArray/Inverter Controller/Voltage Regulator ==
  Vdc_meas : Inport  PortDimensions=1
  Vdc_ref : Inport  Port=2  PortDimensions=1
  Kp : Inport  Port=3  PortDimensions=1
  Ki : Inport  Port=4  PortDimensions=1
  PI regulator with anti-windup D : Subsystem  DialogController=POWERSYS.PowerSysDialog  mask(Discrete PI Controller){Kp=Kp_VDCreg, Ki=Ki_VDCreg, Par_Limits=Limits_VDCreg, Init=0, Ts=Ts}
      mask prompts: Kp "Proportional gain (Kp):"; Ki "Integral gain (Ki):"; Par_Limits "Output limits: [ Upper   Lower ]"; Init "Output initial value:"; Ts "Sample time:"
      mask help: This block implements a discrete PI controller.
      mask init:
      | UpperLimit=Par_Limits(1);
      | LowerLimit=Par_Limits(2);
      | power_initmask();
      mask Help: This block is part of a subset of blocks in the Extras library that does not have documentation associated with it, other than the block mask description.
      mask Display: disp('PI');
  Rtot_pu3 : Gain  Gain=1/Vnom_dc  SaturateOnIntegerOverflow=on  OutDataTypeStr=Inherit: Same as input  ParamDataTypeStr=Inherit: Same as input
  Sum : Sum  Inputs=|+-
  Id_ref : Outport  SampleTime=Ts  InitialOutput=0  VectorParamsAs1DForOutWhenUnconnected=off
  wires:
  Ki/1 -> PI regulator with anti-windup D/3(Ki)
  Kp/1 -> PI regulator with anti-windup D/2(Kp)
  Sum/1 -> Rtot_pu3/1
  Vdc_meas/1 -> Sum/1
  Vdc_ref/1 -> Sum/2
  Rtot_pu3/1 -> PI regulator with anti-windup D/1(Error)
  PI regulator with anti-windup D/1(Out) -> Id_ref/1

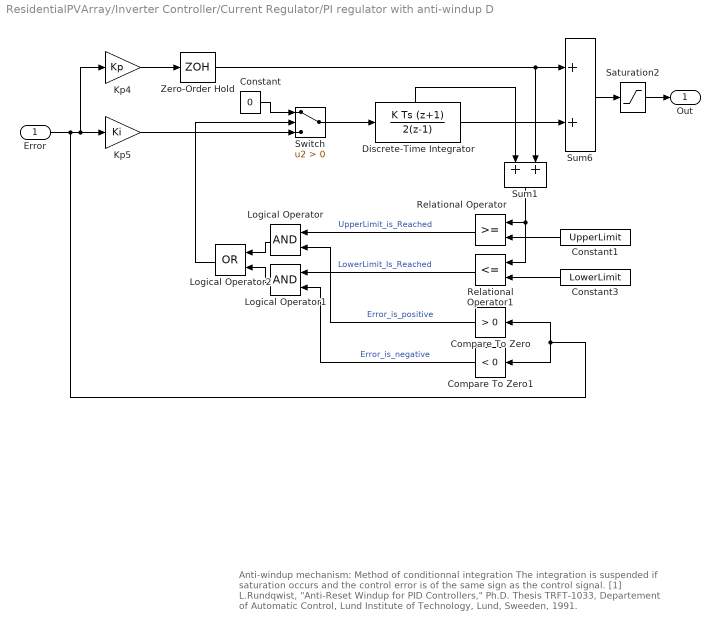
== system ResidentialPVArray/Inverter Controller/Current Regulator/PI regulator with anti-windup D ==
  note: Anti-windup mechanism: Method of conditionnal integration
      |
      | The integration is suspended if saturation occurs and the
      | control error is of the same sign as the control signal.
      |
      | [1] L.Rundqwist, "Anti-Reset Windup for PID Controllers," Ph.D. Thesis TRFT-1033,
      | Departement of Automatic Control, Lund Institute of Technology, Lund, Sweeden, 1991.
  Error : Inport  SampleTime=Ts
  Compare To Zero : simulink/Logic and Bit Operations/Compare To Zero  relop=>  OutDataTypeStr=uint8  ZeroCross=off
  Compare To Zero1 : simulink/Logic and Bit Operations/Compare To Zero  relop=<  OutDataTypeStr=uint8  ZeroCross=off
  Constant : Constant  Value=0
  Constant1 : Constant  Value=UpperLimit
  Constant3 : Constant  Value=LowerLimit
  Discrete-Time Integrator : DiscreteIntegrator  IntegratorMethod=Integration: Trapezoidal  InitialCondition=Init  SampleTime=Ts  LimitOutput=on  UpperSaturationLimit=UpperLimit  LowerSaturationLimit=LowerLimit  ShowStatePort=on  ICPrevOutput=DiscIntNeverNeededParam  ICPrevScaledInput=DiscIntNeverNeededParam
  Kp4 : Gain  Gain=Kp  SaturateOnIntegerOverflow=on  SampleTime=Ts  OutDataTypeStr=Inherit: Same as input  ParamDataTypeStr=Inherit: Same as input
  Kp5 : Gain  Gain=Ki  SaturateOnIntegerOverflow=on  SampleTime=Ts  OutDataTypeStr=Inherit: Same as input  ParamDataTypeStr=Inherit: Same as input
  Logical Operator : Logic  AllPortsSameDT=off  OutDataTypeStr=boolean
  Logical Operator1 : Logic  AllPortsSameDT=off  OutDataTypeStr=boolean
  Logical Operator2 : Logic  Operator=OR  AllPortsSameDT=off  OutDataTypeStr=boolean
  Relational Operator : RelationalOperator  OutDataTypeStr=boolean  InputSameDT=off
  Relational Operator1 : RelationalOperator  Operator=<=  OutDataTypeStr=boolean  InputSameDT=off
  Saturation2 : Saturate  UpperLimit=UpperLimit  LowerLimit=LowerLimit  SampleTime=Ts
  Sum1 : Sum  InputSameDT=on  SaturateOnIntegerOverflow=on  SampleTime=Ts  OutDataTypeStr=Inherit: Same as first input
  Sum6 : Sum  InputSameDT=on  SaturateOnIntegerOverflow=on  SampleTime=Ts  OutDataTypeStr=Inherit: Same as first input
  Switch : Switch  Criteria=u2 > Threshold  SaturateOnIntegerOverflow=off  InputSameDT=off
  Zero-Order Hold : ZeroOrderHold  SampleTime=Ts
  Out : Outport  SampleTime=Ts  InitialOutput=0  VectorParamsAs1DForOutWhenUnconnected=off
  wires:
  Kp5/1 -> Switch/3
  Switch/1 -> Discrete-Time Integrator/1
  Saturation2/1 -> Out/1
  Discrete-Time Integrator/1 -> Sum6/2
  Kp4/1 -> Zero-Order Hold/1
  Sum6/1 -> Saturation2/1
  Error/1 -> Kp5/1, Kp4/1, Compare To Zero/1, Compare To Zero1/1
  Compare To Zero1/1 -> Logical Operator1/2  "Error_is_negative"
  Logical Operator1/1 -> Logical Operator2/2
  Logical Operator/1 -> Logical Operator2/1
  Compare To Zero/1 -> Logical Operator/2  "Error_is_positive"
  Constant3/1 -> Relational Operator1/2
  Constant1/1 -> Relational Operator/2
  Relational Operator1/1 -> Logical Operator1/1  "LowerLimit_Is_Reached"
  Relational Operator/1 -> Logical Operator/1  "UpperLimit_is_Reached"
  Logical Operator2/1 -> Switch/2
  Sum1/1 -> Relational Operator/1, Relational Operator1/1
  Discrete-Time Integrator/State -> Sum1/1
  Zero-Order Hold/1 -> Sum6/1, Sum1/2
  Constant/1 -> Switch/1

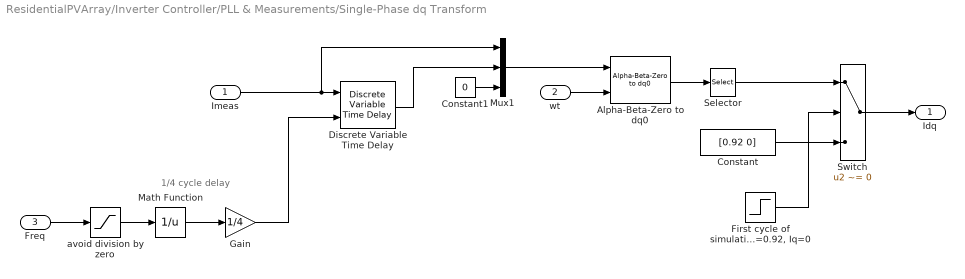
== system ResidentialPVArray/Inverter Controller/PLL & Measurements/Single-Phase dq Transform ==
  note: 1/4 cycle delay
  Imeas : Inport
  wt : Inport  Port=2
  Freq : Inport  Port=3
  Alpha-Beta-Zero to dq0 : spsAlphaBetaZerotodq0Lib/Alpha-Beta-Zero to dq0  Alignment=90 degrees behind phase A axis
  Constant : Constant  Value=[0.92 0]
  Constant1 : Constant  Value=0
  Discrete Variable Time Delay : spsDiscreteVariableTimeDelayLib/Discrete Variable Time Delay  MaxDelay=1  InitialValue=0  Ts=Ts  DFT=on
  "First cycle of simulation Id=0.92, Iq=0" : Step  Time=1/Fnom  SampleTime=Ts
  Gain : Gain  Gain=1/4
  Math Function : Math  Operator=reciprocal  SignedPower=on
  Mux1 : Mux  Inputs=3
  Selector : Selector  InputPortWidth=3  IndexOptions=Index vector (dialog)  Indices=[1 2]  OutputSizes=1
  Switch : Switch  Criteria=u2 ~= 0  SaturateOnIntegerOverflow=off  InputSameDT=off
  avoid division by zero : Saturate  UpperLimit=70  LowerLimit=40
  Idq : Outport  VectorParamsAs1DForOutWhenUnconnected=off
  wires:
  "First cycle of simulation Id=0.92, Iq=0"/1 -> Switch/2
  Constant/1 -> Switch/3
  Switch/1 -> Idq/1
  Selector/1 -> Switch/1
  Gain/1 -> Discrete Variable Time Delay/2
  Math Function/1 -> Gain/1
  avoid division by zero/1 -> Math Function/1
  Freq/1 -> avoid division by zero/1
  Alpha-Beta-Zero to dq0/1 -> Selector/1
  wt/1 -> Alpha-Beta-Zero to dq0/2
  Imeas/1 -> Mux1/1, Discrete Variable Time Delay/1
  Mux1/1 -> Alpha-Beta-Zero to dq0/1
  Discrete Variable Time Delay/1 -> Mux1/2
  Constant1/1 -> Mux1/3

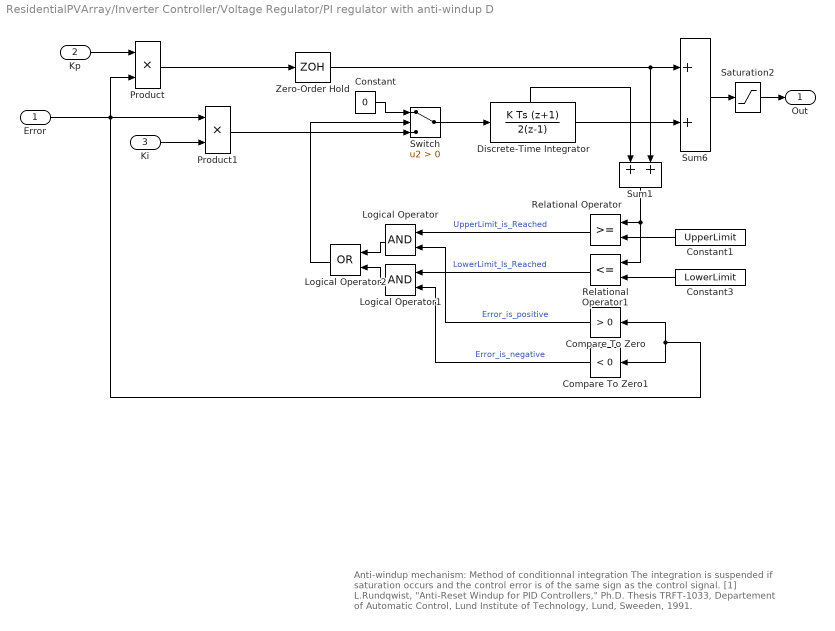
== system ResidentialPVArray/Inverter Controller/Voltage Regulator/PI regulator with anti-windup D ==
  note: Anti-windup mechanism: Method of conditionnal integration
      |
      | The integration is suspended if saturation occurs and the
      | control error is of the same sign as the control signal.
      |
      | [1] L.Rundqwist, "Anti-Reset Windup for PID Controllers," Ph.D. Thesis TRFT-1033,
      | Departement of Automatic Control, Lund Institute of Technology, Lund, Sweeden, 1991.
  Error : Inport  SampleTime=Ts
  Kp : Inport  Port=2  SampleTime=Ts
  Ki : Inport  Port=3  SampleTime=Ts
  Compare To Zero : simulink/Logic and Bit Operations/Compare To Zero  relop=>  OutDataTypeStr=uint8  ZeroCross=off
  Compare To Zero1 : simulink/Logic and Bit Operations/Compare To Zero  relop=<  OutDataTypeStr=uint8  ZeroCross=off
  Constant : Constant  Value=0
  Constant1 : Constant  Value=UpperLimit
  Constant3 : Constant  Value=LowerLimit
  Discrete-Time Integrator : DiscreteIntegrator  IntegratorMethod=Integration: Trapezoidal  InitialCondition=Init  SampleTime=Ts  LimitOutput=on  UpperSaturationLimit=UpperLimit  LowerSaturationLimit=LowerLimit  ShowStatePort=on  ICPrevOutput=DiscIntNeverNeededParam  ICPrevScaledInput=DiscIntNeverNeededParam
  Logical Operator : Logic  AllPortsSameDT=off  OutDataTypeStr=boolean
  Logical Operator1 : Logic  AllPortsSameDT=off  OutDataTypeStr=boolean
  Logical Operator2 : Logic  Operator=OR  AllPortsSameDT=off  OutDataTypeStr=boolean
  Product : Product
  Product1 : Product
  Relational Operator : RelationalOperator  OutDataTypeStr=boolean  InputSameDT=off
  Relational Operator1 : RelationalOperator  Operator=<=  OutDataTypeStr=boolean  InputSameDT=off
  Saturation2 : Saturate  UpperLimit=UpperLimit  LowerLimit=LowerLimit  SampleTime=Ts
  Sum1 : Sum  InputSameDT=on  SaturateOnIntegerOverflow=on  SampleTime=Ts  OutDataTypeStr=Inherit: Same as first input
  Sum6 : Sum  InputSameDT=on  SaturateOnIntegerOverflow=on  SampleTime=Ts  OutDataTypeStr=Inherit: Same as first input
  Switch : Switch  Criteria=u2 > Threshold  SaturateOnIntegerOverflow=off  InputSameDT=off
  Zero-Order Hold : ZeroOrderHold  SampleTime=Ts
  Out : Outport  SampleTime=Ts  InitialOutput=0  VectorParamsAs1DForOutWhenUnconnected=off
  wires:
  Ki/1 -> Product1/2
  Kp/1 -> Product/1
  Product1/1 -> Switch/3
  Switch/1 -> Discrete-Time Integrator/1
  Saturation2/1 -> Out/1
  Discrete-Time Integrator/1 -> Sum6/2
  Product/1 -> Zero-Order Hold/1
  Sum6/1 -> Saturation2/1
  Error/1 -> Product1/1, Product/2, Compare To Zero/1, Compare To Zero1/1
  Compare To Zero1/1 -> Logical Operator1/2  "Error_is_negative"
  Logical Operator1/1 -> Logical Operator2/2
  Logical Operator/1 -> Logical Operator2/1
  Compare To Zero/1 -> Logical Operator/2  "Error_is_positive"
  Constant3/1 -> Relational Operator1/2
  Constant1/1 -> Relational Operator/2
  Relational Operator1/1 -> Logical Operator1/1  "LowerLimit_Is_Reached"
  Relational Operator/1 -> Logical Operator/1  "UpperLimit_is_Reached"
  Logical Operator2/1 -> Switch/2
  Sum1/1 -> Relational Operator/1, Relational Operator1/1
  Discrete-Time Integrator/State -> Sum1/1
  Zero-Order Hold/1 -> Sum6/1, Sum1/2
  Constant/1 -> Switch/1

== matlab function ResidentialPVArray/MPPT Controller/MPPT Control ==
  settings: updateMethod=DISCRETE  sampleTime=Ts
  data: V input =V; I input; D output; Dmax parameter; Dmin parameter; deltaD parameter; Dinit parameter; Scan_On input; DeltaD_Scan parameter
function D   = PandO(V, I, Dmax, Dmin, deltaD, Dinit, Scan_On, DeltaD_Scan)

% MPPT controller based on the Perturb & Observe algorithm.

% D output = Duty cycle of the boost converter (value between 0 and 1)
% V input = PV array terminal voltage (V)
% I input = PV array current (A)
% D = 1 - Vinput/Voutput (increasing D decrease Vin)

persistent Vold Pold Dold Scan_On_Old Pmax D_Pmax V_Pmax;
%
if isempty(Vold)
    Vold=0;
    Pold=0;
    Scan_On_Old=0;
    Dold=Dinit;
    Pmax=0;
    D_Pmax=0;
    V_Pmax=0;
end
P= V*I;
if Scan_On==1 || Scan_On_Old==1
    if Scan_On_Old==0
        Scan_On_Old=1;
        D=Dmin;
    else
        D=Dold+DeltaD_Scan;
    end
    Dold=D;
    if P>Pmax
        Pmax=P;
        D_Pmax=D;
    end
    if D >= Dmax
        Scan_On_Old=0;
        Pold=Pmax;
        Dold=D_Pmax;
        Vold=V_Pmax;
    end
else
    dV= V - Vold;
    dP= P - Pold;
    %
    if dP ~= 0
        if dP < 0
            if dV < 0
                D = Dold - deltaD;
            else
                D = Dold + deltaD;
            end
        else
            if dV < 0
                D = Dold + deltaD;
            else
                D = Dold - deltaD;
            end
        end
    else
        D=Dold;
    end
    %
    if D >= Dmax || D<= Dmin
        D=Dold;
    end
    %
    Dold=D;
    Vold=V;
    Pold=P;
end
